simulink library "mlib_301825"  (Simulink 6.5)
settings Model: Creator=mshakeri  LastModifiedBy=mshakeri  ExtModeAutoUpdateStatusClock=off

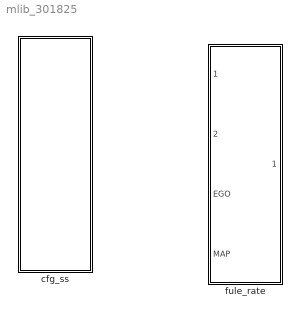
== system mlib_301825 ==
  cfg_ss : Subsystem
      settings: TemplateBlock=self
  fule_rate : Subsystem  TreatAsAtomicUnit=on

== system mlib_301825/cfg_ss ==

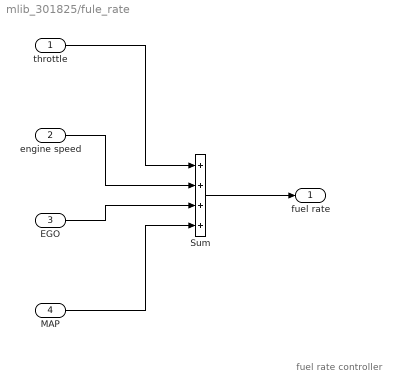
== system mlib_301825/fule_rate ==
  note: fuel rate controller
  throttle : Inport  SampleTime=.01
  engine speed : Inport  Port=2  SampleTime=.01
  EGO : Inport  Port=3  SampleTime=.01
  MAP : Inport  Port=4  SampleTime=.01
  Sum : Sum  Inputs=++++
  fuel rate : Outport  InitialOutput=0
  wires:
  Sum/1 -> fuel rate/1
  MAP/1 -> Sum/4
  EGO/1 -> Sum/3
  engine speed/1 -> Sum/2
  throttle/1 -> Sum/1
